simulink model "PI_EMS"  (R2022b)
settings: Solver=VariableStepAuto  StartTime=0.0  StopTime=10.0  RelTol=1e-6
values from neighbouring files (symbols this model uses):
  current_filter_order = 20    [bancada_1gdl.m]
  diferent_values = (2^N)-1    (= 65535)    [bancada_1gdl.m]
  f_current_control = 2000    [bancada_1gdl.m]
  fl_current = 10000    [bancada_1gdl.m]
  fs_current = 20000    [bancada_1gdl.m]
  kd_current = 0    [bancada_1gdl.m]
  offset_current = 0.001065378087271    (= 0.00106537808727)    [bancada_1gdl.m]
  suelo = 25/1000    (= 0.025)    [bancada_1gdl.m]    (also in graficasLevitacion.m = 619.512; graphs_corporativas.m = 620.5614)
  var_current = 0.052125100064495    (= 0.0521251000645)    [bancada_1gdl.m]
undefined symbols (not defined in the file or in its folder): DiscIntNeverNeededParam
libraries: simulink x1
settings Model: Creator=ramuj  LastModifiedBy=ramuj

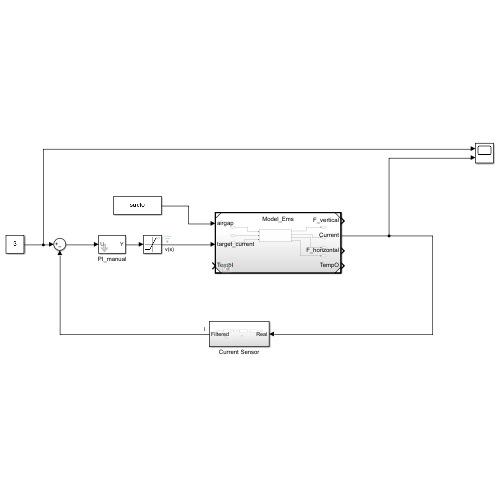
[thumbnail: Simulink's stored preview of the top-level diagram]
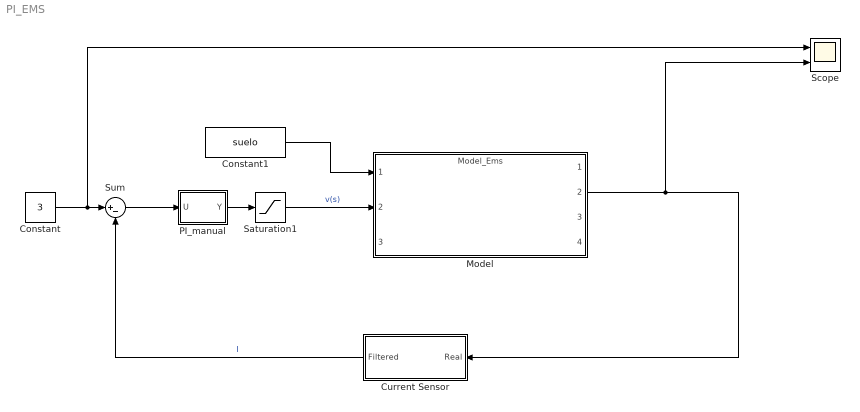
== system PI_EMS ==
  Constant : Constant  Value=3
  Constant1 : Constant  Value=suelo
  Current Sensor : Subsystem
  Model : ModelReference  ModelNameDialog=Model_Ems.slx  SimulationMode=Normal  ModelReferenceVersion=1.23
  PI_manual : Subsystem  mask{Kp=50, Ki=400, Kd=kd_current, N=kd_current, f=f_current_control}
  Saturation1 : Saturate  UpperLimit=100*0.8  LowerLimit=-100*0.8
  Scope : Scope  NumInputPorts=2
  Sum : Sum  Inputs=|+-
  wires:
  Saturation1/1 -> Model/2  "v(s)"
  PI_manual/1(Y) -> Saturation1/1
  Constant1/1 -> Model/1
  Constant/1 -> Scope/1, Sum/1
  Sum/1 -> PI_manual/1(U)
  Model/2 -> Scope/2, Current Sensor/1(Real)
  Current Sensor/1(Filtered) -> Sum/2  "I"

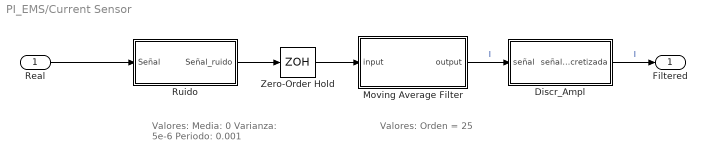
== system PI_EMS/Current Sensor ==
  note: Valores:
      | Media: 0
      | Varianza: 5e-6
      | Periodo: 0.001
  note: Valores:
      | Orden = 25
  Real : Inport
  Discr_Ampl : Subsystem  mask{N=diferent_values, Min=-50, Max=50}
      mask prompts: N "Valores distintos (N)"; Min "Valor mínimo"; Max "Valor máximo"
      mask DialogControl DescGroupVar Prompt: Discretizacion_Amplitud
      mask DialogControl DescTextVar Prompt: Discretización en amplitud
  Moving Average Filter : Subsystem  mask{M=current_filter_order, fs=-1}
      mask prompts: M "Orden del filtro (M)"; fs "Frecuencia de muestreo (fs)"
  Ruido : Subsystem  mask{M=offset_current, V=var_current, T=1/fs_current}
      mask prompts: M "Media"; V "Varianza"; T "Periodo"
      mask DialogControl Ruido Prompt: Ruido
      mask DialogControl DescTextVar Prompt: Añade ruido gaussiano
  Zero-Order Hold : ZeroOrderHold  SampleTime=1/fl_current
  Filtered : Outport
  wires:
  Real/1 -> Ruido/1(Señal)
  Discr_Ampl/1(señal_discretizada) -> Filtered/1  "I"
  Moving Average Filter/1(output) -> Discr_Ampl/1(señal)  "I"
  Ruido/1(Señal_ruido) -> Zero-Order Hold/1
  Zero-Order Hold/1 -> Moving Average Filter/1(input)

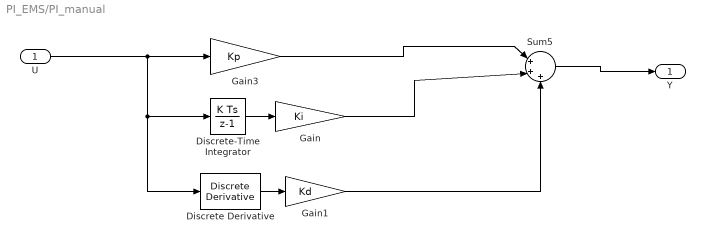
== system PI_EMS/PI_manual ==
  U : Inport
  Discrete Derivative : simulink/Discrete/Discrete Derivative  gainval=1.0  ICPrevScaledInput=0  OutMin=[]  OutMax=[]  OutDataType=fixdt(1, 16)  OutScaling=2^-10  DoSatur=off
  Discrete-Time Integrator : DiscreteIntegrator  SampleTime=1/f  ICPrevOutput=DiscIntNeverNeededParam  ICPrevScaledInput=DiscIntNeverNeededParam
  Gain : Gain  Gain=Ki
  Gain1 : Gain  Gain=Kd
  Gain3 : Gain  Gain=Kp
  Sum5 : Sum  Inputs=|+++
  Y : Outport
  wires:
  Discrete Derivative/1 -> Gain1/1
  Gain1/1 -> Sum5/3
  Gain/1 -> Sum5/2
  Discrete-Time Integrator/1 -> Gain/1
  Gain3/1 -> Sum5/1
  U/1 -> Discrete Derivative/1, Discrete-Time Integrator/1, Gain3/1
  Sum5/1 -> Y/1

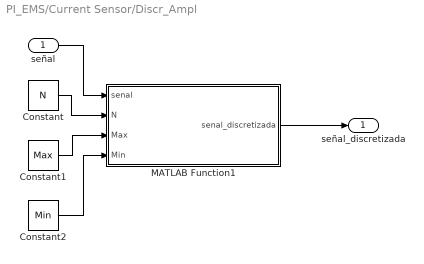
== system PI_EMS/Current Sensor/Discr_Ampl ==
  señal : Inport
  Constant : Constant  Value=N
  Constant1 : Constant  Value=Max
  Constant2 : Constant  Value=Min
  MATLAB Function1 : MATLAB Function  TreatAsAtomicUnit=on
  señal_discretizada : Outport
  wires:
  MATLAB Function1/1(senal_discretizada) -> señal_discretizada/1
  señal/1 -> MATLAB Function1/1(senal)
  Constant1/1 -> MATLAB Function1/3(Max)
  Constant/1 -> MATLAB Function1/2(N)
  Constant2/1 -> MATLAB Function1/4(Min)

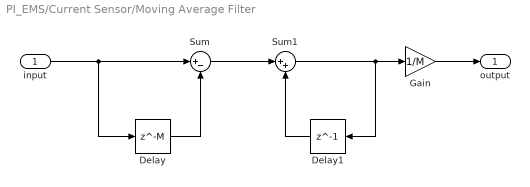
== system PI_EMS/Current Sensor/Moving Average Filter ==
  input : Inport
  Delay : Delay  DelayLength=M  SampleTime=fs
  Delay1 : Delay  DelayLength=1  SampleTime=fs
  Gain : Gain  Gain=1/M
  Sum : Sum  Inputs=|+-
  Sum1 : Sum  Inputs=|++
  output : Outport
  wires:
  input/1 -> Delay/1, Sum/1
  Delay/1 -> Sum/2
  Sum/1 -> Sum1/1
  Sum1/1 -> Delay1/1, Gain/1
  Delay1/1 -> Sum1/2
  Gain/1 -> output/1

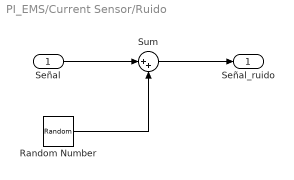
== system PI_EMS/Current Sensor/Ruido ==
  Señal : Inport
  Random Number : RandomNumber  Mean=M  Variance=V  Seed=3  SampleTime=T
  Sum : Sum  Inputs=|++
  Señal_ruido : Outport
  wires:
  Random Number/1 -> Sum/2
  Señal/1 -> Sum/1
  Sum/1 -> Señal_ruido/1

== matlab function PI_EMS/Current Sensor/Discr_Ampl/MATLAB Function1 ==
  data: senal input; senal_discretizada output; N input; Max input; Min input
function senal_discretizada  = fcn(senal,N,Max,Min)

if(senal>Max)
    senal_discretizada=Max;
    return
elseif(senal<Min)
    senal_discretizada=Min;
    return
end

valor_escalon=(Max-Min)/(N-1);
i=Min;
 while(i<Max)
    if(i+valor_escalon/2>senal)
        senal_discretizada=i;
        return
    end
    i=i+valor_escalon;
end

      senal_discretizada=Max;
end
